simulink model "sih"  (R2026a)
settings: Solver=VariableStepAuto  StopTime=240000
undefined symbols (not defined in the file or in its folder): m, n
settings Model: Creator=tsvd  LastModifiedBy=tsvd

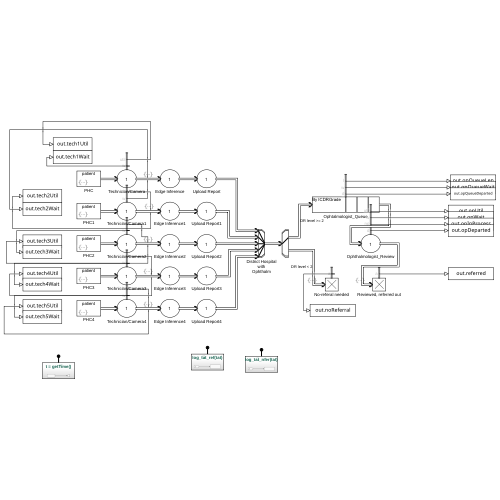
[thumbnail: Simulink's stored preview of the top-level diagram]
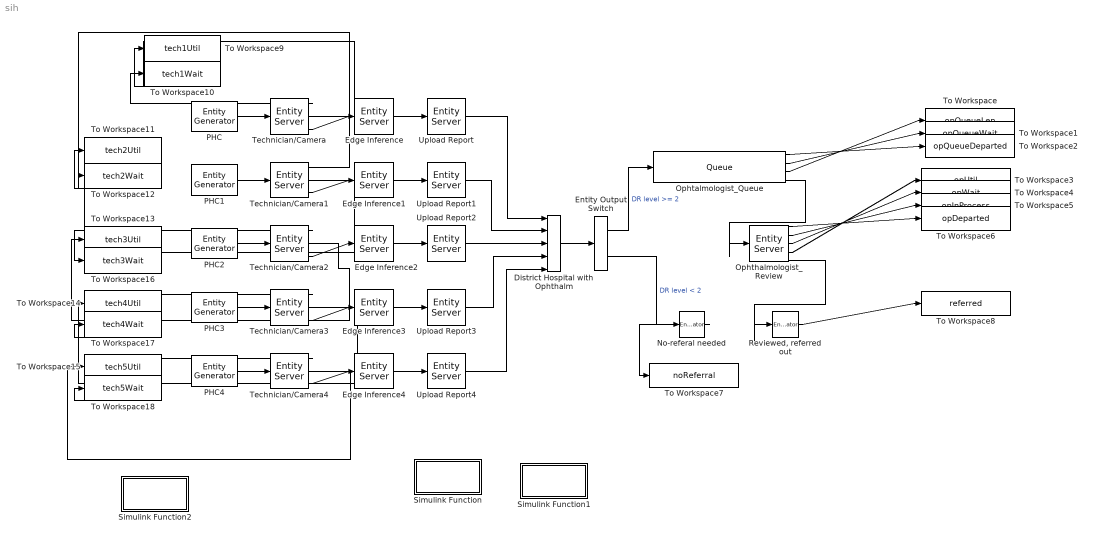
== system sih ==
  District Hospital with Ophthalm : EntityInputSwitch  InputPortMessageModes=m,m,m,m,m  OutputPortMessageModes=m  NumberInputPorts=5
      settings: InputPortMap=u1,u2,u3,u4,u5
  Edge Inference : EntityServer  InputPortMessageModes=m  OutputPortMessageModes=m  Capacity=1  EntryAction=|
      | w = [168 25 168 93 62];
      | cw = cumsum(w)/sum(w);
      | r = rand;
      | g = sum(r > cw);
      | entity.ICDRGrade = g;
      | if entity.ICDRGrade >= 2
      |     entity.referralPort = 1;
      | else
      |     entity.referralPort = 2;
      | end
  Edge Inference1 : EntityServer  InputPortMessageModes=m  OutputPortMessageModes=m  Capacity=1  EntryAction=|
      | w = [168 25 168 93 62];
      | cw = cumsum(w)/sum(w);
      | r = rand;
      | g = sum(r > cw);
      | entity.ICDRGrade = g;
      | if entity.ICDRGrade >= 2
      |     entity.referralPort = 1;
      | else
      |     entity.referralPort = 2;
      | end
  Edge Inference2 : EntityServer  InputPortMessageModes=m  OutputPortMessageModes=m  Capacity=1  EntryAction=|
      | w = [168 25 168 93 62];
      | cw = cumsum(w)/sum(w);
      | r = rand;
      | g = sum(r > cw);
      | entity.ICDRGrade = g;
      | if entity.ICDRGrade >= 2
      |     entity.referralPort = 1;
      | else
      |     entity.referralPort = 2;
      | end
  Edge Inference3 : EntityServer  InputPortMessageModes=m  OutputPortMessageModes=m  Capacity=1  EntryAction=|
      | w = [168 25 168 93 62];
      | cw = cumsum(w)/sum(w);
      | r = rand;
      | g = sum(r > cw);
      | entity.ICDRGrade = g;
      | if entity.ICDRGrade >= 2
      |     entity.referralPort = 1;
      | else
      |     entity.referralPort = 2;
      | end
  Edge Inference4 : EntityServer  InputPortMessageModes=m  OutputPortMessageModes=m  Capacity=1  EntryAction=|
      | w = [168 25 168 93 62];
      | cw = cumsum(w)/sum(w);
      | r = rand;
      | g = sum(r > cw);
      | entity.ICDRGrade = g;
      | if entity.ICDRGrade >= 2
      |     entity.referralPort = 1;
      | else
      |     entity.referralPort = 2;
      | end
  Entity Output Switch : EntityOutputSwitch  InputPortMessageModes=m  OutputPortMessageModes=m,m  SwitchingCriterion=From attribute  SwitchAttributeName=referralPort
  No-referal needed : EntityTerminator  InputPortMessageModes=m  EntryAction=|  NumberEntitiesArrived=on
      | entity.tat = getTime() - entity.genTime;
      | log_tat_ref(entity.tat);
      settings: OutputPortMap=o0
  Ophtalmologist_Queue : Queue  InputPortMessageModes=m  OutputPortMessageModes=n,n,n,m  Capacity=Inf  QueueType=Priority  PrioritySource=ICDRGrade  SortingDirection=Descending  NumberEntitiesDeparted=on  AverageWait=on  AverageQueueLength=on
      settings: OutputPortMap=o0,o2,o3,o5
  Ophthalmologist_Review : EntityServer  InputPortMessageModes=m  OutputPortMessageModes=n,n,n,n,m  Capacity=1  ServiceTimeValue=2  NumberEntitiesDeparted=on  NumberEntitiesPending=on  AverageWait=on  Utilization=on
      settings: OutputPortMap=o0,o3,o4,o5,o9
  PHC{,1..4} (5 alike) : EntityGenerator  OutputPortMessageModes=m  Period=12  GenerateAction=entity.genTime = getTime();  AttributeName=ICDRGrade|referralPort|genTime|tat  AttributeInitialValue=0|1|0|0  EntityType=Structured  EntityTypeName=patient
  "Reviewed, referred out" : EntityTerminator  InputPortMessageModes=m  EntryAction=|  NumberEntitiesArrived=on
      | entity.tat = getTime() - entity.genTime;
      | log_tat_nfer(entity.tat);
      settings: OutputPortMap=o0
  Simulink Function : Subsystem  TreatAsAtomicUnit=on
  Simulink Function1 : Subsystem  TreatAsAtomicUnit=on
  Simulink Function2 : Subsystem  TreatAsAtomicUnit=on
  Technician/Camera{,1..4} (5 alike) : EntityServer  InputPortMessageModes=m  OutputPortMessageModes=n,n,m  Capacity=1  ServiceTimeValue=5 + (rand < 0.15)*5  AverageWait=on  Utilization=on
      settings: OutputPortMap=o4,o5,o9
  To Workspace : ToWorkspace  VariableName=opQueueLen  SaveFormat=Timeseries  SampleTime=-1
  To Workspace1 : ToWorkspace  VariableName=opQueueWait  SaveFormat=Timeseries  SampleTime=-1
  To Workspace10 : ToWorkspace  VariableName=tech1Wait  SaveFormat=Timeseries  SampleTime=-1
  To Workspace11 : ToWorkspace  VariableName=tech2Util  SaveFormat=Timeseries  SampleTime=-1
  To Workspace12 : ToWorkspace  VariableName=tech2Wait  SaveFormat=Timeseries  SampleTime=-1
  To Workspace13 : ToWorkspace  VariableName=tech3Util  SaveFormat=Timeseries  SampleTime=-1
  To Workspace14 : ToWorkspace  VariableName=tech4Util  SaveFormat=Timeseries  SampleTime=-1
  To Workspace15 : ToWorkspace  VariableName=tech5Util  SaveFormat=Timeseries  SampleTime=-1
  To Workspace16 : ToWorkspace  VariableName=tech3Wait  SaveFormat=Timeseries  SampleTime=-1
  To Workspace17 : ToWorkspace  VariableName=tech4Wait  SaveFormat=Timeseries  SampleTime=-1
  To Workspace18 : ToWorkspace  VariableName=tech5Wait  SaveFormat=Timeseries  SampleTime=-1
  To Workspace2 : ToWorkspace  VariableName=opQueueDeparted  SaveFormat=Timeseries  SampleTime=-1
  To Workspace3 : ToWorkspace  VariableName=opUtil  SaveFormat=Timeseries  SampleTime=-1
  To Workspace4 : ToWorkspace  VariableName=opWait  SaveFormat=Timeseries  SampleTime=-1
  To Workspace5 : ToWorkspace  VariableName=opInProcess  SaveFormat=Timeseries  SampleTime=-1
  To Workspace6 : ToWorkspace  VariableName=opDeparted  SaveFormat=Timeseries  SampleTime=-1
  To Workspace7 : ToWorkspace  VariableName=noReferral  SaveFormat=Timeseries  SampleTime=-1
  To Workspace8 : ToWorkspace  VariableName=referred  SaveFormat=Timeseries  SampleTime=-1
  To Workspace9 : ToWorkspace  VariableName=tech1Util  SaveFormat=Timeseries  SampleTime=-1
  Upload Report{,1..4} (5 alike) : EntityServer  InputPortMessageModes=m  OutputPortMessageModes=m  Capacity=1  ServiceTimeValue=0.3
  wires:
  PHC/1 -> Technician/Camera/1
  Technician/Camera/3 -> Edge Inference/1
  Edge Inference/1 -> Upload Report/1
  Upload Report/1 -> District Hospital with Ophthalm/1
  District Hospital with Ophthalm/1 -> Entity Output Switch/1
  Technician/Camera1/3 -> Edge Inference1/1
  Edge Inference1/1 -> Upload Report1/1
  Technician/Camera2/3 -> Edge Inference2/1
  Edge Inference2/1 -> Upload Report2/1
  Technician/Camera3/3 -> Edge Inference3/1
  Edge Inference3/1 -> Upload Report3/1
  Technician/Camera4/3 -> Edge Inference4/1
  Edge Inference4/1 -> Upload Report4/1
  Upload Report1/1 -> District Hospital with Ophthalm/2
  Upload Report2/1 -> District Hospital with Ophthalm/3
  Upload Report3/1 -> District Hospital with Ophthalm/4
  Upload Report4/1 -> District Hospital with Ophthalm/5
  Entity Output Switch/1 -> Ophtalmologist_Queue/1  "DR level >= 2"
  Entity Output Switch/2 -> No-referal needed/1  "DR level < 2"
  Ophtalmologist_Queue/4 -> Ophthalmologist_Review/1
  Ophthalmologist_Review/5 -> "Reviewed, referred out"/1
  Ophtalmologist_Queue/3 -> To Workspace/1
  Ophtalmologist_Queue/2 -> To Workspace1/1
  Ophtalmologist_Queue/1 -> To Workspace2/1
  Ophthalmologist_Review/1 -> To Workspace6/1
  Ophthalmologist_Review/2 -> To Workspace5/1
  Ophthalmologist_Review/3 -> To Workspace4/1
  Ophthalmologist_Review/4 -> To Workspace3/1
  No-referal needed/1 -> To Workspace7/1
  "Reviewed, referred out"/1 -> To Workspace8/1
  Technician/Camera/2 -> To Workspace9/1
  Technician/Camera/1 -> To Workspace10/1
  Technician/Camera1/2 -> To Workspace11/1
  Technician/Camera1/1 -> To Workspace12/1
  Technician/Camera2/1 -> To Workspace16/1
  Technician/Camera2/2 -> To Workspace13/1
  Technician/Camera3/1 -> To Workspace17/1
  Technician/Camera3/2 -> To Workspace14/1
  Technician/Camera4/1 -> To Workspace18/1
  Technician/Camera4/2 -> To Workspace15/1
  PHC1/1 -> Technician/Camera1/1
  PHC2/1 -> Technician/Camera2/1
  PHC3/1 -> Technician/Camera3/1
  PHC4/1 -> Technician/Camera4/1

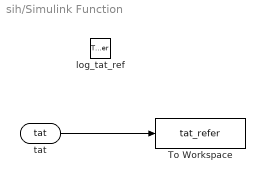
== system sih/Simulink Function ==
  log_tat_ref : TriggerPort  TriggerType=function-call  IsSimulinkFunction=on  FunctionName=log_tat_ref  FunctionVisibility=scoped  VariantControl=(inherit)
  To Workspace : ToWorkspace  VariableName=tat_refer  SaveFormat=Timeseries  SampleTime=-1
  tat : ArgIn  DisableCoverage=on  ArgumentName=tat
  wires:
  tat/1 -> To Workspace/1

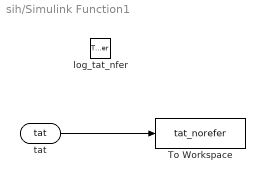
== system sih/Simulink Function1 ==
  log_tat_nfer : TriggerPort  TriggerType=function-call  IsSimulinkFunction=on  FunctionName=log_tat_nfer  FunctionVisibility=scoped  VariantControl=(inherit)
  To Workspace : ToWorkspace  VariableName=tat_norefer  SaveFormat=Timeseries  SampleTime=-1
  tat : ArgIn  DisableCoverage=on  ArgumentName=tat
  wires:
  tat/1 -> To Workspace/1

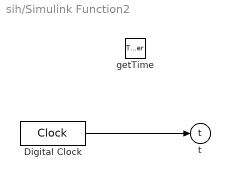
== system sih/Simulink Function2 ==
  getTime : TriggerPort  TriggerType=function-call  IsSimulinkFunction=on  FunctionName=getTime  FunctionVisibility=scoped  VariantControl=(inherit)
  Digital Clock : DigitalClock  SampleTime=-1
  t : ArgOut  ArgumentName=t
  wires:
  Digital Clock/1 -> t/1
